simulink model "Controller"  (R2020b)
settings: Solver=FixedStepDiscrete  StartTime=0.0  StopTime=20  FixedStep=1e-4  RelTol=1e-3
settings Model: DataDictionary=pid.sldd  Creator=The MathWorks, Inc.  LastModifiedBy=moody
settings DataIOCC: SaveFormat=Array
settings OptimizationCC: DefaultParameterBehavior=Inlined  UseDivisionForNetSlopeComputation=on  GainParamInheritBuiltInType=on  UseFloatMulNetSlope=on  InlineInvariantSignals=on  ExpressionDepthLimit=2147483647  EfficientFloat2IntCast=on  LifeSpan=1  EfficientTunableParamExpr=on
settings DebuggingCC: SolverPrmCheckMsg=warning  UniqueDataStoreMsg=error  AssertControl=DisableAll  AllowSymbolicDim=off  ModelReferenceSymbolNameMessage=none  StateNameClashWarn=warning  StrictBusMsg=ErrorOnBusTreatedAsVector  SFUnexpectedBacktrackingDiag=warning  SFNoUnconditionalDefaultTransitionDiag=warning  SFExecutionAtInitializationDiag=none  ArithmeticOperatorsInVariantConditions=warning
settings HardwareCC: ProdBitPerPointer=32  ProdBitPerSizeT=32  ProdBitPerPtrDiffT=32  ProdLargestAtomicInteger=Long  ProdLargestAtomicFloat=Double  ProdWordSize=32  ProdHWDeviceType=ARM Compatible->ARM Cortex-M
settings ModelReferenceCC: PropagateSignalLabelsOutOfModel=off
settings SFSimCC: SimUseLocalCustomCode=off  CustomCodeUndefinedFunction=UseInterfaceOnly
settings RTWCC: Description=Embedded Coder  SystemTargetFile=ert.tlc  GenCodeOnly=on  TemplateMakefile=ert_default_tmf  GenerateReport=on  RTWUseLocalCustomCode=off  IncludeHyperlinkInReport=on  GenerateTraceInfo=on  GenerateTraceReport=on  GenerateTraceReportSl=on  GenerateTraceReportSf=on  GenerateTraceReportEml=on  GenerateCodeMetricsReport=on
settings CodeAppCC: IgnoreCustomStorageClasses=off  IgnoreTestpoints=on  CustomSymbolStrType=$N$R$M  StateflowObjectComments=on  InternalIdentifier=Classic
settings ERTTargetCC: MultiwordLength=2048  GenerateSampleERTMain=on  CodeInterfacePackaging=Reusable function  SupportNonFinite=off  InlinedParameterPlacement=NonHierarchical  RootIOFormat=Structure reference  ERTSrcFileBannerTemplate=code_c_template.cgt  ERTHdrFileBannerTemplate=code_h_template.cgt  ERTDataSrcFileTemplate=data_c_template.cgt  ERTDataHdrFileTemplate=data_h_template.cgt  ERTCustomFileTemplate=example_file_process.tlc  ERTFilePackagingFormat=Compact  RateTransitionBlockCode=Function  ConvertIfToSwitch=off  SuppressUnreachableDefaultCases=off
settings ConfigComp: CovEnable=on  CovScope=Subsystem  RecordCoverage=on  CovPath=Controller  CovMetricSettings=dcmw  CovEnableCumulative=off  CovSaveCumulativeToWorkspaceVar=on  CovSaveSingleToWorkspaceVar=on  CovExternalEMLEnable=off  CovSFcnEnable=off

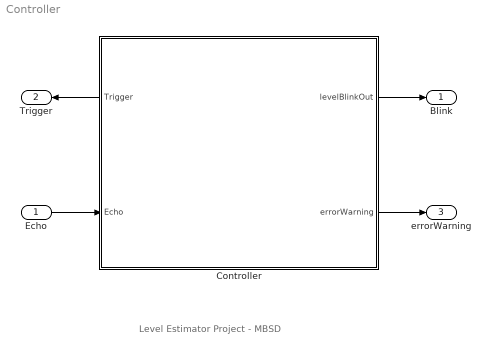
== system Controller ==
  note: Level Estimator Project - MBSD
  Echo : Inport  OutDataTypeStr=boolean  PortDimensions=1
  Controller : Subsystem
      settings: PortSchema="{\"entries\":[{\"content\":{\"sides\":[{\"content\":{\"connectorIds\":[\"Out3\",\"In1\"]},\"type\":\"ConnectorPlacement.EquallySpacedRectSide\",\"uuid\":\"a3d0d6f9-f622-4308-87ee-c57e45fbb6e4\"},{\"content\":{\"connectorIds\":[\"Out1\",\"Out2\"],\"side\":\"RIGHT\"},\"type\":\"ConnectorPlacement.EquallySpacedRectSide\",\"uuid\":\"a5ea927a-a6f2-4562-b679-61b475a8fbe4\"},{\"content\":{\"connectorIds\":[],\"side\":\"TOP\"},\"type\":\"ConnectorPlacement.EquallySpacedRectSide\",\"uuid\":\"1e637b39-b9a5-4f12-82b5-ed0355b5accd\"},{\"content\":{\"connectorIds\":[],\"side\":\"HIDDEN\"},\"type\":\"ConnectorPlacement.EquallySpacedRectSide\",\"uuid\":\"250e11c3-0ed0-404f-93aa-d91786cbeb3a\"}]},\"type\":\"ConnectorPlacement.EquallySpacedConnector\",\"uuid\":\"6d409785-a54a-4a37-a2b5-766043901591\"}],\"packageUris\":[\"http://schema.mathworks.com/mf0/Connector/R2020b\"],\"version\":\"1.0\"}"
  Blink : Outport
  Trigger : Outport  Port=2  OutDataTypeStr=boolean  PortDimensions=1
  errorWarning : Outport  Port=3
  wires:
  Controller/1(levelBlinkOut) -> Blink/1
  Controller/3(Trigger) -> Trigger/1
  Controller/2(errorWarning) -> errorWarning/1
  Echo/1 -> Controller/1(Echo)

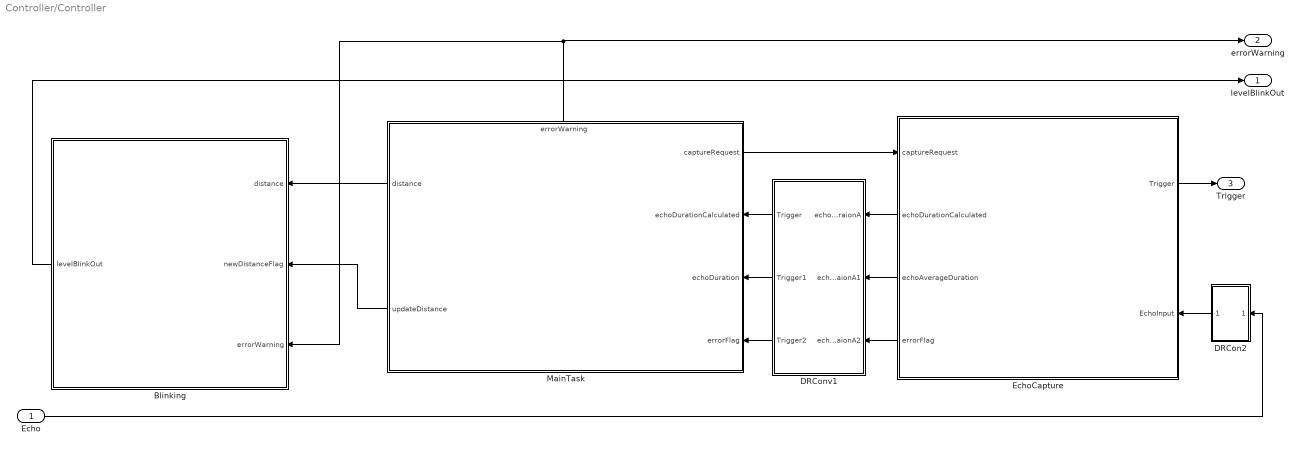
== system Controller/Controller ==
  Echo : Inport
  Blinking : Stateflow chart  TreatAsAtomicUnit=on
  DRCon2 : Subsystem
  DRConv1 : Subsystem
  EchoCapture : Stateflow chart  TreatAsAtomicUnit=on
      settings: PortSchema="{\"entries\":[{\"content\":{\"sides\":[{\"content\":{\"connectorIds\":[\"In2\",\"Out2\",\"Out3\",\"Out4\"]},\"type\":\"ConnectorPlacement.EquallySpacedRectSide\",\"uuid\":\"b640a457-5908-42ca-a248-f55ab2a74d55\"},{\"content\":{\"connectorIds\":[\"Out1\",\"In1\"],\"side\":\"RIGHT\"},\"type\":\"ConnectorPlacement.EquallySpacedRectSide\",\"uuid\":\"16f6f838-3691-4317-97bf-b76eedcf1803\"},{\"content\":{\"connectorIds\":[],\"side\":\"TOP\"},\"type\":\"ConnectorPlacement.EquallySpacedRectSide\",\"uuid\":\"d1d48549-b82e-49cc-957d-fd6911d427cc\"},{\"content\":{\"connectorIds\":[],\"side\":\"HIDDEN\"},\"type\":\"ConnectorPlacement.EquallySpacedRectSide\",\"uuid\":\"54c5d872-2f74-4312-a114-225f36180143\"}]},\"type\":\"ConnectorPlacement.EquallySpacedConnector\",\"uuid\":\"02c5b3a5-a0c3-468c-8271-92f881ee808b\"}],\"packageUris\":[\"http://schema.mathworks.com/mf0/Connector/R2020b\"],\"version\":\"1.0\"}"
  MainTask : Stateflow chart  TreatAsAtomicUnit=on
      settings: PortSchema="{\"entries\":[{\"content\":{\"sides\":[{\"content\":{\"connectorIds\":[\"Out1\",\"In1\",\"In2\",\"In3\"]},\"type\":\"ConnectorPlacement.EquallySpacedRectSide\",\"uuid\":\"171e6474-a786-4c2b-b8c7-77d26b5a77c4\"},{\"content\":{\"connectorIds\":[\"Out2\",\"Out3\"],\"side\":\"RIGHT\"},\"type\":\"ConnectorPlacement.EquallySpacedRectSide\",\"uuid\":\"d084a4c6-6e19-4253-b0f6-c9e34142edc7\"},{\"content\":{\"connectorIds\":[\"Out4\"],\"side\":\"TOP\"},\"type\":\"ConnectorPlacement.EquallySpacedRectSide\",\"uuid\":\"3a29a072-8ba5-47a2-b7c6-829758876f8f\"},{\"content\":{\"connectorIds\":[],\"side\":\"HIDDEN\"},\"type\":\"ConnectorPlacement.EquallySpacedRectSide\",\"uuid\":\"947af842-f7da-4608-a9d3-74e4c8c49916\"}]},\"type\":\"ConnectorPlacement.EquallySpacedConnector\",\"uuid\":\"e4d5997a-2644-4bab-8288-c8bde8f0fc77\"}],\"packageUris\":[\"http://schema.mathworks.com/mf0/Connector/R2020b\"],\"version\":\"1.0\"}"
  levelBlinkOut : Outport
  errorWarning : Outport  Port=2
  Trigger : Outport  Port=3
  wires:
  MainTask/4(errorWarning) -> errorWarning/1, Blinking/3(errorWarning)
  DRConv1/1(Trigger) -> MainTask/1(echoDurationCalculated)
  DRConv1/2(Trigger1) -> MainTask/2(echoDuration)
  DRCon2/1(Trigger) -> EchoCapture/1(EchoInput)
  EchoCapture/2(echoDurationCalculated) -> DRConv1/1(echoDuraionA)
  EchoCapture/3(echoAverageDuration) -> DRConv1/2(echoDuraionA1)
  MainTask/1(captureRequest) -> EchoCapture/2(captureRequest)
  EchoCapture/1(Trigger) -> Trigger/1
  EchoCapture/4(errorFlag) -> DRConv1/3(echoDuraionA2)
  DRConv1/3(Trigger2) -> MainTask/3(errorFlag)
  Blinking/1(levelBlinkOut) -> levelBlinkOut/1
  Echo/1 -> DRCon2/1(In1)
  MainTask/2(distance) -> Blinking/1(distance)
  MainTask/3(updateDistance) -> Blinking/2(newDistanceFlag)

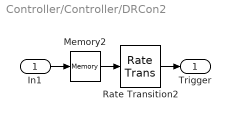
== system Controller/Controller/DRCon2 ==
  In1 : Inport
  Memory2 : Memory
  Rate Transition2 : RateTransition
  Trigger : Outport
  wires:
  Rate Transition2/1 -> Trigger/1
  In1/1 -> Memory2/1
  Memory2/1 -> Rate Transition2/1

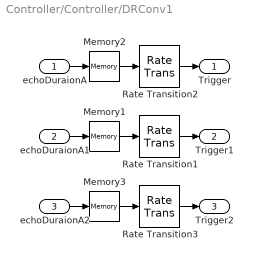
== system Controller/Controller/DRConv1 ==
  echoDuraionA : Inport
  echoDuraionA1 : Inport  Port=2
  echoDuraionA2 : Inport  Port=3
  Memory1 : Memory
  Memory2 : Memory
  Memory3 : Memory
  Rate Transition1 : RateTransition
  Rate Transition2 : RateTransition
  Rate Transition3 : RateTransition
  Trigger : Outport
  Trigger1 : Outport  Port=2
  Trigger2 : Outport  Port=3
  wires:
  Rate Transition2/1 -> Trigger/1
  echoDuraionA/1 -> Memory2/1
  Memory2/1 -> Rate Transition2/1
  Rate Transition1/1 -> Trigger1/1
  echoDuraionA1/1 -> Memory1/1
  Memory1/1 -> Rate Transition1/1
  Rate Transition3/1 -> Trigger2/1
  echoDuraionA2/1 -> Memory3/1
  Memory3/1 -> Rate Transition3/1

== stateflow chart Controller/Blinking ==
  settings: initializeOutput=1
  state Blinking [parallel]
    settings: executionOrder=2
    state StateOn
      levelBlinkOut = true;
    state StateOff
      levelBlinkOut = false;
    (default) -> StateOn
    StateOff -> StateOn : after(offTime,msec)
    StateOn -> StateOff : [after(onTime,msec)...
        |  && onTime ~= 100]
  state updateDistance [parallel]
    settings: executionOrder=1
    state startState
      blinkBasedOnDistance(distance)
    state blinkBasedOnDistance(distanceIn) [function]
      (default) -> (junction 178) : % decide blinkTaskIndex based on distance
      (junction 178) -> (junction 179) [order 1] : [ distanceIn >= 10 && distanceIn <= 100 ]
      (junction 178) -> (junction 180) [order 2]
      (junction 179) -> (junction 184) : {onTime = uint16(distanceIn); offTime = uint16(100-distanceIn);}
      (junction 180) -> (junction 181) [order 1] : [distanceIn > 3 && distanceIn < 10]
      (junction 180) -> (junction 211) [order 2]
      (junction 181) -> (junction 183) : {onTime = 250; offTime = 250;}
      (junction 211) -> (junction 214) [order 1] : [distanceIn >  100 &&  distanceIn <= 400]
      (junction 211) -> (junction 182) [order 2] : {onTime = 500; offTime = 500;}
      (junction 214) -> (junction 215) : {onTime = 250; offTime = 250;}
      (junction 215) -> (junction 182)
      (junction 183) -> (junction 215)
      (junction 184) -> (junction 183)
      (junction 182) -> (junction 185)
    (default) -> startState
    startState -> startState : [newDistanceFlag == true || errorWarning == true]
  data: distanceIn function_input; distance input double size=1; levelBlinkOut output boolean size=1 =false; newDistanceFlag input boolean size=1 =false; errorWarning input boolean size=1; offTime local uint16 size=1 =uint16(0); onTime local uint16 size=1 =uint16(0)

== stateflow chart Controller/EchoCapture ==
  state EchoDurationCapture [parallel]
    settings: executionOrder=1
    state waitingCaptureRequest
      entry:
      counter = 0;
      errorFlag = false;
      exit:
      echoDurationCalculated = false;
      echoAverageDuration = 0;
    state calculateDurationAverage
      entry:
      echoAverageDuration = ...
      echoAverageDuration/4;
      echoDurationCalculated = true;
    state triggerOn
      entry:
      Trigger = true;
      exit:
      Trigger = false
      counter = counter+1;
    state chech_N_Trigger
    state echoError
      entry:
      counter = 0;
      errorFlag =  true;
    state checkEchoOn
      entry, during, exit:
      echoOffDuraion = elapsed(msec);
    state calculateEchoDuration
      entry, during, exit:
      echoOnDuraion = elapsed(usec);
    state exitState
      entry:
      echoAverageDuration = ...
      echoAverageDuration + echoOnDuraion;
    (default) -> waitingCaptureRequest
    (junction 542) -> waitingCaptureRequest
    calculateDurationAverage -> waitingCaptureRequest
    (junction 540) -> (junction 542) : after(30, msec)
    waitingCaptureRequest -> triggerOn : [captureRequest == true]
    chech_N_Trigger -> calculateDurationAverage [order 1] : [counter >= 4]
    (junction 537) -> triggerOn : after(30, msec)
    echoError -> (junction 537)
    chech_N_Trigger -> triggerOn [order 2] : after(30, msec)
    triggerOn -> checkEchoOn : after(10, msec)
    (junction 429) -> chech_N_Trigger
    checkEchoOn -> echoError [order 2] : [echoOffDuraion > 3]
    checkEchoOn -> calculateEchoDuration [order 1] : [EchoInput == true]
    calculateEchoDuration -> (junction 540) [order 1] : [errorFlag ==  true]
    calculateEchoDuration -> exitState [order 2] : [EchoInput == false &&  errorFlag == false]
    exitState -> (junction 429)
  data: Trigger output boolean =false; EchoInput input; counter local uint8 =uint8(0); captureRequest input boolean size=1; echoDurationCalculated output boolean size=1 =false; echoAverageDuration output double size=1 =0; errorFlag output boolean size=1 =false; echoOffDuraion local; echoOnDuraion local

== stateflow chart Controller/MainTask ==
  state mainTask [parallel]
    settings: executionOrder=1
    state InitialState
      entry:
      captureRequest = false;
      updateDistance = false;
    state waitingErrorHandler
      entry:
      distance = 0;
      errorWarning = true;
      exit:
      errorWarning = false;
    state requestOn
      entry:
      captureRequest = true;
    state requestOff
      entry:
      captureRequest = false;
    state DistanceCalcualtion
      entry:
      updateDistance = true;
      distance = echoDuration/58;
    state CalcualtionexitState
      entry:
      updateDistance = false;
    state waitWakeUp
      taskCompleted = true
    (default) -> InitialState
    waitingErrorHandler -> InitialState : [errorFlag == false]
    (junction 83) -> InitialState
    (junction 82) -> (junction 83)
    InitialState -> requestOn
    (junction 42) -> waitingErrorHandler
    requestOn -> requestOff
    requestOff -> (junction 42) [order 2] : [errorFlag == true]
    requestOff -> DistanceCalcualtion [order 1] : [echoDurationCalculated == true]
    DistanceCalcualtion -> CalcualtionexitState
    CalcualtionexitState -> waitWakeUp
    waitWakeUp -> (junction 82) : [taskCompleted == false]
  state wakeEvery1sec [parallel]
    settings: executionOrder=2
    state wait1sec
    state clearTaskComoleted
      taskCompleted = false
    (default) -> wait1sec
    clearTaskComoleted -> wait1sec
    wait1sec -> clearTaskComoleted : after(1000, msec)
  data: captureRequest output boolean size=1 =false; echoDurationCalculated input boolean size=1; distance output double size=1; updateDistance output boolean size=1 =false; echoDuration input double size=1; errorFlag input boolean size=1; errorWarning output boolean size=1 =false; taskCompleted local boolean size=1 =false
